simulink model "BPSK_Rayleigh_FLAT_FLAT"  (R2021a)
settings: Solver=VariableStepAuto  StartTime=0.0  StopTime=Inf  RelTol=1e-3
undefined symbols (not defined in the file or in its folder): gaussian
libraries: commdigbbndpm3 x2, simulink x2, commchan3 x1, commrandsrc3 x1, commsink2 x1
settings Model: Creator=roberto  LastModifiedBy=roberto

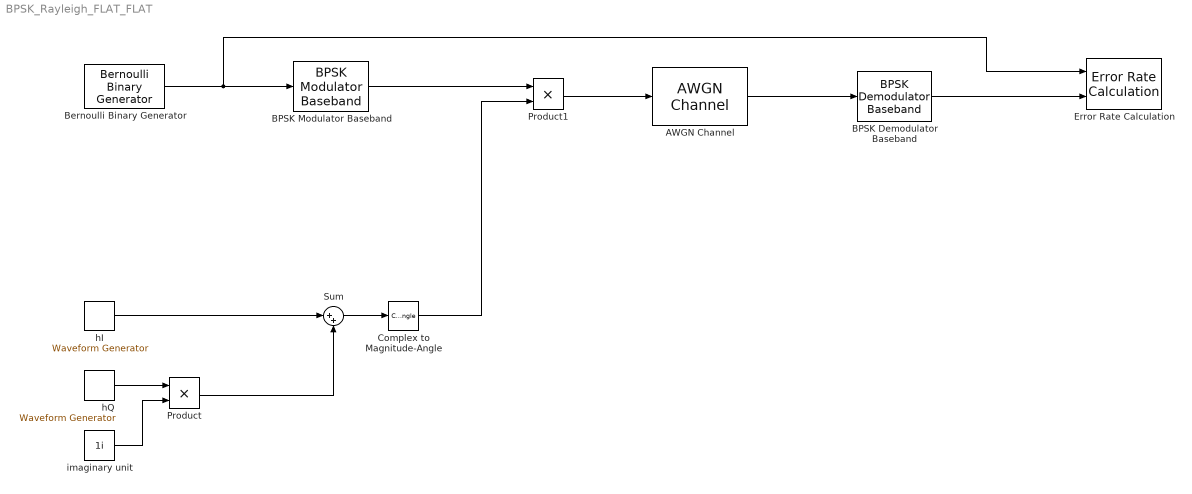
== system BPSK_Rayleigh_FLAT_FLAT ==
  AWGN Channel : commchan3/AWGN Channel  InputProcessing=Columns as channels (frame based)  seed=67  noiseMode="Signal to noise ratio  (Eb/No)"  EbNodB=EbNo  EsNodB=10  SNRdB=10  bitsPerSym=1  Ps=1  Tsym=1  variance=1
  BPSK Demodulator Baseband : commdigbbndpm3/BPSK Demodulator Baseband  DecType=Hard decision  VarSource=Dialog  Variance=1  Ph=0  outDtype=Inherit via internal rule  derotateFactorWordLen=16  derotateFactorDataTypeStr=Inherit: Same word length as input  derotateFactorLastDataTypeStr=Inherit: Same word length as input
  BPSK Modulator Baseband : commdigbbndpm3/BPSK Modulator Baseband  Ph=0  outDtype=double  outWordLen=16  outUDDataType=sfix(16)  outFracLenMode=Best precision  outFracLen=15  outDataTypeStr=double  outLastDataTypeStr=double
  Bernoulli Binary Generator : commrandsrc3/Bernoulli Binary Generator  ProbabilityOfZero=0.5  SeedSource=Auto  Seed=0  SampleTime=1  SamplesPerFrame=1  OutputDataType=double  SimulateUsing=Interpreted execution
  Complex to Magnitude-Angle : ComplexToMagnitudeAngle  Output=Magnitude
  Error Rate Calculation : commsink2/Error Rate Calculation  N=0  st_delay=0  cp_mode=Entire frame  subframe=[]  PMode=Workspace  WsName=ErrorVec0  RsMode2=off  stop=on  numErr=maxNumErrs  maxBits=maxNumBits
  Product : Product
  Product1 : Product
  Sum : Sum  Inputs=|++
  hI : simulink/Sources/Waveform Generator  OutMin=[]  OutMax=[]  OutDataTypeStr=double  SelectedSignal=1  Signals=gaussian('Mean',0,'Variance',0.5,'Seed',1)  BlockNames=MultiportSwitch_fb556a3493b141a  SampleTime=1
  hQ : simulink/Sources/Waveform Generator  OutMin=[]  OutMax=[]  OutDataTypeStr=double  SelectedSignal=1  Signals=gaussian('Mean',0,'Variance',0.5,'Seed',67)  BlockNames=MultiportSwitch_47572b58e7994c6  SampleTime=1
  imaginary unit : Constant  Value=1i
  wires:
  Bernoulli Binary Generator/1 -> Error Rate Calculation/1, BPSK Modulator Baseband/1
  AWGN Channel/1 -> BPSK Demodulator Baseband/1
  BPSK Demodulator Baseband/1 -> Error Rate Calculation/2
  hQ/1 -> Product/1
  Product1/1 -> AWGN Channel/1
  BPSK Modulator Baseband/1 -> Product1/1
  imaginary unit/1 -> Product/2
  Product/1 -> Sum/2
  hI/1 -> Sum/1
  Sum/1 -> Complex to Magnitude-Angle/1
  Complex to Magnitude-Angle/1 -> Product1/2
